simulink model "IEEE_9bus_v2_"  (Simulink 8.4)
settings: Solver=ode4  StartTime=0.0  StopTime=inf  FixedStep=Ts  RelTol=1e-3
PostLoadFcn:
  | Ts=25e-6;Rs=5*1.867;cs=1.4080e-004;
InitFcn:
  | Ts=25e-6;Rs=5*1.867;cs=1.4080e-004;
undefined symbols (not defined in the file): another_event_name, DiscIntNeverNeededParam, gcbh, my_event_name, sps_rtmsupport
libraries: powerlib x36, spsVIMeasurementModel x27, library x9, rtlab x4, artemis x3, sps_avr x3
(part 2 of 2)

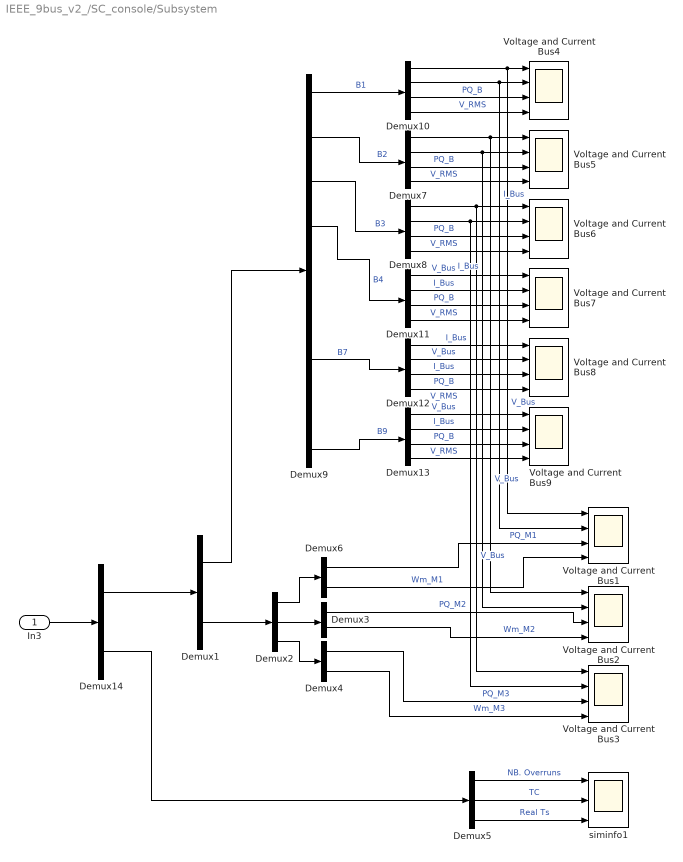
== system IEEE_9bus_v2_/SC_console/Subsystem ==
  In3 : Inport
  Demux1 : Demux  Outputs=[99 9]
  Demux{7..8,10..13} (6 alike) : Demux  Outputs=[3 3 2 3]
  Demux14 : Demux  Outputs=[108 3]
  Demux2 : Demux  Outputs=3
  Demux3 : Demux  Outputs=[2 1]
  Demux4 : Demux  Outputs=[2 1]
  Demux5 : Demux  Outputs=3
  Demux6 : Demux  Outputs=[2 1]
  Demux9 : Demux  Outputs=[11 11 11 11 11 11 11 11 11]
  Voltage and Current Bus{1..9} (9 alike) : Scope  NumInputPorts=4
      Voltage and Current Bus1 settings: TimeRange=0.1  MaxDataPoints=15000  SaveToWorkspace=off  SaveName=mach10  YMin=-1.25~-0.75~-0.5~1  YMax=1.25~0.75~0.3~1.00001  SampleTime=-1
      Voltage and Current Bus2 settings: TimeRange=0.1  MaxDataPoints=15000  SaveToWorkspace=off  SaveName=mach11  YMin=-1.25~-0.75~-0.5~1  YMax=1.25~0.75~0.3~1.00001  SampleTime=-1
      Voltage and Current Bus3 settings: TimeRange=0.1  MaxDataPoints=15000  SaveToWorkspace=off  SaveName=mach12  YMin=-1.25~-0.75~-0.5~1  YMax=1.25~0.75~0.3~1.00001  SampleTime=-1
      Voltage and Current Bus4 settings: TimeRange=0.1  LimitDataPoints=on  MaxDataPoints=15000  SaveToWorkspace=off  SaveName=mach13  YMin=-1~-0.9~-0.8~-5  YMax=1~0.9~0.5~5  SampleTime=-1
      Voltage and Current Bus5 settings: TimeRange=0.1  LimitDataPoints=on  MaxDataPoints=15000  SaveToWorkspace=off  SaveName=mach  YMin=-1~-0.9~-0.8~-5  YMax=1~0.9~0.5~5  SampleTime=-1
      Voltage and Current Bus6 settings: TimeRange=0.1  LimitDataPoints=on  MaxDataPoints=15000  SaveToWorkspace=off  SaveName=mach1  YMin=-1~-0.9~-0.8~-5  YMax=1~0.9~0.5~5  SampleTime=-1
      Voltage and Current Bus7 settings: TimeRange=0.1  LimitDataPoints=on  MaxDataPoints=15000  SaveToWorkspace=off  SaveName=mach3  YMin=-1~-0.9~-0.8~-5  YMax=1~0.9~0.5~5  SampleTime=-1
      Voltage and Current Bus8 settings: TimeRange=0.1  LimitDataPoints=on  MaxDataPoints=15000  SaveToWorkspace=off  SaveName=mach4  YMin=-1~-0.9~-0.8~-5  YMax=1~0.9~0.5~5  SampleTime=-1
      Voltage and Current Bus9 settings: TimeRange=0.1  LimitDataPoints=on  MaxDataPoints=15000  SaveToWorkspace=off  SaveName=mach5  YMin=-1~-0.9~-0.8~-5  YMax=1~0.9~0.5~5  SampleTime=-1
  siminfo1 : Scope  NumInputPorts=3
      settings: TimeRange=0.8  LimitDataPoints=on  MaxDataPoints=15000  SaveToWorkspace=off  SaveName=mach2  YMin=-1~-1~-1  YMax=1~1~1  SampleTime=-1
  wires:
  Demux5/3 -> siminfo1/3  "Real Ts"
  Demux5/1 -> siminfo1/1  "NB. Overruns"
  Demux5/2 -> siminfo1/2  "TC"
  Demux3/2 -> Voltage and Current Bus2/4  "Wm_M2"
  Demux2/1 -> Demux6/1
  Demux6/1 -> Voltage and Current Bus1/3  "PQ_M1"
  Demux1/2 -> Demux2/1
  Demux4/2 -> Voltage and Current Bus3/4  "Wm_M3"
  Demux4/1 -> Voltage and Current Bus3/3  "PQ_M3"
  Demux3/1 -> Voltage and Current Bus2/3  "PQ_M2"
  Demux2/2 -> Demux3/1
  Demux2/3 -> Demux4/1
  Demux6/2 -> Voltage and Current Bus1/4  "Wm_M1"
  Demux1/1 -> Demux9/1
  Demux9/1 -> Demux10/1  "B1"
  Demux10/1 -> Voltage and Current Bus1/1, Voltage and Current Bus4/1  "V_Bus"
  Demux10/2 -> Voltage and Current Bus1/2, Voltage and Current Bus4/2  "I_Bus"
  Demux10/3 -> Voltage and Current Bus4/3  "PQ_B"
  In3/1 -> Demux14/1
  Demux14/2 -> Demux5/1
  Demux14/1 -> Demux1/1
  Demux10/4 -> Voltage and Current Bus4/4  "V_RMS"
  Demux7/1 -> Voltage and Current Bus2/1, Voltage and Current Bus5/1  "V_Bus"
  Demux7/2 -> Voltage and Current Bus2/2, Voltage and Current Bus5/2  "I_Bus"
  Demux7/3 -> Voltage and Current Bus5/3  "PQ_B"
  Demux7/4 -> Voltage and Current Bus5/4  "V_RMS"
  Demux8/1 -> Voltage and Current Bus3/1, Voltage and Current Bus6/1  "V_Bus"
  Demux8/2 -> Voltage and Current Bus3/2, Voltage and Current Bus6/2  "I_Bus"
  Demux8/3 -> Voltage and Current Bus6/3  "PQ_B"
  Demux8/4 -> Voltage and Current Bus6/4  "V_RMS"
  Demux11/1 -> Voltage and Current Bus7/1  "V_Bus"
  Demux11/2 -> Voltage and Current Bus7/2  "I_Bus"
  Demux11/3 -> Voltage and Current Bus7/3  "PQ_B"
  Demux11/4 -> Voltage and Current Bus7/4  "V_RMS"
  Demux12/1 -> Voltage and Current Bus8/1  "V_Bus"
  Demux12/2 -> Voltage and Current Bus8/2  "I_Bus"
  Demux12/3 -> Voltage and Current Bus8/3  "PQ_B"
  Demux12/4 -> Voltage and Current Bus8/4  "V_RMS"
  Demux13/1 -> Voltage and Current Bus9/1  "V_Bus"
  Demux13/2 -> Voltage and Current Bus9/2  "I_Bus"
  Demux13/3 -> Voltage and Current Bus9/3  "PQ_B"
  Demux13/4 -> Voltage and Current Bus9/4  "V_RMS"
  Demux9/2 -> Demux7/1  "B2"
  Demux9/3 -> Demux8/1  "B3"
  Demux9/4 -> Demux11/1  "B4"
  Demux9/7 -> Demux12/1  "B7"
  Demux9/9 -> Demux13/1  "B9"

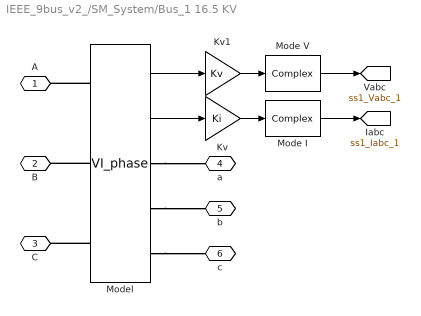
== system IEEE_9bus_v2_/SM_System/Bus_1 16.5 KV ==
  Kv : Gain  Gain=Ki  SaturateOnIntegerOverflow=on  OutDataTypeStr=Inherit: Same as input  ParamDataTypeStr=Inherit: Same as input
  Kv1 : Gain  Gain=Kv  SaturateOnIntegerOverflow=on  OutDataTypeStr=Inherit: Same as input  ParamDataTypeStr=Inherit: Same as input
  Mode I : spsVIMeasurementModel/Complex
  Mode V : spsVIMeasurementModel/Complex
  Model : spsVIMeasurementModel/VI_phase  SystemSampleTime=-1
  A : PMIOPort  Port=1  Side=Left
  B : PMIOPort  Port=2  Side=Left
  C : PMIOPort  Port=3  Side=Left
  a : PMIOPort  Port=4  Side=Right
  b : PMIOPort  Port=5  Side=Right
  c : PMIOPort  Port=6  Side=Right
  tag scope: ss1_Iabc_1=global, ss1_Vabc_1=global
  wires:
  Model/2 -> Kv/1
  Model/1 -> Kv1/1
  Kv/1 -> Mode I/1
  Kv1/1 -> Mode V/1
  Mode I/1 -> [ss1_Iabc_1]
  Mode V/1 -> [ss1_Vabc_1]
  connections:
  Model/RConn3 -- c/RConn1
  Model/RConn1 -- a/RConn1
  Model/RConn2 -- b/RConn1
  Model/LConn3 -- C/RConn1
  Model/LConn1 -- A/RConn1
  Model/LConn2 -- B/RConn1

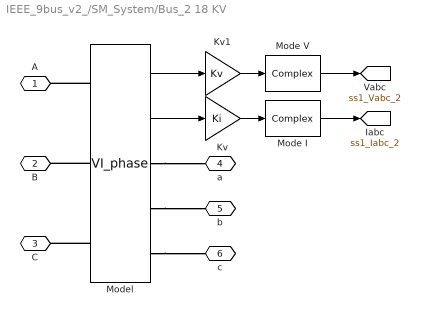
== system IEEE_9bus_v2_/SM_System/Bus_2 18 KV ==
  Kv : Gain  Gain=Ki  SaturateOnIntegerOverflow=on  OutDataTypeStr=Inherit: Same as input  ParamDataTypeStr=Inherit: Same as input
  Kv1 : Gain  Gain=Kv  SaturateOnIntegerOverflow=on  OutDataTypeStr=Inherit: Same as input  ParamDataTypeStr=Inherit: Same as input
  Mode I : spsVIMeasurementModel/Complex
  Mode V : spsVIMeasurementModel/Complex
  Model : spsVIMeasurementModel/VI_phase  SystemSampleTime=-1
  A : PMIOPort  Port=1  Side=Left
  B : PMIOPort  Port=2  Side=Left
  C : PMIOPort  Port=3  Side=Left
  a : PMIOPort  Port=4  Side=Right
  b : PMIOPort  Port=5  Side=Right
  c : PMIOPort  Port=6  Side=Right
  tag scope: ss1_Iabc_2=global, ss1_Vabc_2=global
  wires:
  Model/2 -> Kv/1
  Model/1 -> Kv1/1
  Kv/1 -> Mode I/1
  Kv1/1 -> Mode V/1
  Mode I/1 -> [ss1_Iabc_2]
  Mode V/1 -> [ss1_Vabc_2]
  connections:
  Model/RConn3 -- c/RConn1
  Model/RConn1 -- a/RConn1
  Model/RConn2 -- b/RConn1
  Model/LConn3 -- C/RConn1
  Model/LConn1 -- A/RConn1
  Model/LConn2 -- B/RConn1

== system IEEE_9bus_v2_/SM_System/Bus_3 13.8 KV ==
  Kv : Gain  Gain=Ki  SaturateOnIntegerOverflow=on  OutDataTypeStr=Inherit: Same as input  ParamDataTypeStr=Inherit: Same as input
  Kv1 : Gain  Gain=Kv  SaturateOnIntegerOverflow=on  OutDataTypeStr=Inherit: Same as input  ParamDataTypeStr=Inherit: Same as input
  Mode I : spsVIMeasurementModel/Complex
  Mode V : spsVIMeasurementModel/Complex
  Model : spsVIMeasurementModel/VI_phase  SystemSampleTime=-1
  A : PMIOPort  Port=1  Side=Left
  B : PMIOPort  Port=2  Side=Left
  C : PMIOPort  Port=3  Side=Left
  a : PMIOPort  Port=4  Side=Right
  b : PMIOPort  Port=5  Side=Right
  c : PMIOPort  Port=6  Side=Right
  tag scope: ss1_Iabc_3=global, ss1_Vabc_3=global
  wires:
  Model/2 -> Kv/1
  Model/1 -> Kv1/1
  Kv/1 -> Mode I/1
  Kv1/1 -> Mode V/1
  Mode I/1 -> [ss1_Iabc_3]
  Mode V/1 -> [ss1_Vabc_3]
  connections:
  Model/RConn3 -- c/RConn1
  Model/RConn1 -- a/RConn1
  Model/RConn2 -- b/RConn1
  Model/LConn3 -- C/RConn1
  Model/LConn1 -- A/RConn1
  Model/LConn2 -- B/RConn1

== system IEEE_9bus_v2_/SM_System/Bus_4 230 KV ==
  Kv : Gain  Gain=Ki  SaturateOnIntegerOverflow=on  OutDataTypeStr=Inherit: Same as input  ParamDataTypeStr=Inherit: Same as input
  Kv1 : Gain  Gain=Kv  SaturateOnIntegerOverflow=on  OutDataTypeStr=Inherit: Same as input  ParamDataTypeStr=Inherit: Same as input
  Mode I : spsVIMeasurementModel/Complex
  Mode V : spsVIMeasurementModel/Complex
  Model : spsVIMeasurementModel/VI_phase  SystemSampleTime=-1
  A : PMIOPort  Port=1  Side=Left
  B : PMIOPort  Port=2  Side=Left
  C : PMIOPort  Port=3  Side=Left
  a : PMIOPort  Port=4  Side=Right
  b : PMIOPort  Port=5  Side=Right
  c : PMIOPort  Port=6  Side=Right
  tag scope: ss1_Iabc_4=global, ss1_Vabc_4=global
  wires:
  Model/2 -> Kv/1
  Model/1 -> Kv1/1
  Kv/1 -> Mode I/1
  Kv1/1 -> Mode V/1
  Mode I/1 -> [ss1_Iabc_4]
  Mode V/1 -> [ss1_Vabc_4]
  connections:
  Model/RConn3 -- c/RConn1
  Model/RConn1 -- a/RConn1
  Model/RConn2 -- b/RConn1
  Model/LConn3 -- C/RConn1
  Model/LConn1 -- A/RConn1
  Model/LConn2 -- B/RConn1

== system IEEE_9bus_v2_/SM_System/Bus_5 230 KV ==
  Kv : Gain  Gain=Ki  SaturateOnIntegerOverflow=on  OutDataTypeStr=Inherit: Same as input  ParamDataTypeStr=Inherit: Same as input
  Kv1 : Gain  Gain=Kv  SaturateOnIntegerOverflow=on  OutDataTypeStr=Inherit: Same as input  ParamDataTypeStr=Inherit: Same as input
  Mode I : spsVIMeasurementModel/Complex
  Mode V : spsVIMeasurementModel/Complex
  Model : spsVIMeasurementModel/VI_phase  SystemSampleTime=-1
  A : PMIOPort  Port=1  Side=Left
  B : PMIOPort  Port=2  Side=Left
  C : PMIOPort  Port=3  Side=Left
  a : PMIOPort  Port=4  Side=Right
  b : PMIOPort  Port=5  Side=Right
  c : PMIOPort  Port=6  Side=Right
  tag scope: ss1_Iabc_5=global, ss1_Vabc_5=global
  wires:
  Model/2 -> Kv/1
  Model/1 -> Kv1/1
  Kv/1 -> Mode I/1
  Kv1/1 -> Mode V/1
  Mode I/1 -> [ss1_Iabc_5]
  Mode V/1 -> [ss1_Vabc_5]
  connections:
  Model/RConn3 -- c/RConn1
  Model/RConn1 -- a/RConn1
  Model/RConn2 -- b/RConn1
  Model/LConn3 -- C/RConn1
  Model/LConn1 -- A/RConn1
  Model/LConn2 -- B/RConn1

== system IEEE_9bus_v2_/SM_System/Bus_6 230 KV ==
  Kv : Gain  Gain=Ki  SaturateOnIntegerOverflow=on  OutDataTypeStr=Inherit: Same as input  ParamDataTypeStr=Inherit: Same as input
  Kv1 : Gain  Gain=Kv  SaturateOnIntegerOverflow=on  OutDataTypeStr=Inherit: Same as input  ParamDataTypeStr=Inherit: Same as input
  Mode I : spsVIMeasurementModel/Complex
  Mode V : spsVIMeasurementModel/Complex
  Model : spsVIMeasurementModel/VI_phase  SystemSampleTime=-1
  A : PMIOPort  Port=1  Side=Left
  B : PMIOPort  Port=2  Side=Left
  C : PMIOPort  Port=3  Side=Left
  a : PMIOPort  Port=4  Side=Right
  b : PMIOPort  Port=5  Side=Right
  c : PMIOPort  Port=6  Side=Right
  tag scope: ss1_Iabc_6=global, ss1_Vabc_6=global
  wires:
  Model/2 -> Kv/1
  Model/1 -> Kv1/1
  Kv/1 -> Mode I/1
  Kv1/1 -> Mode V/1
  Mode I/1 -> [ss1_Iabc_6]
  Mode V/1 -> [ss1_Vabc_6]
  connections:
  Model/RConn3 -- c/RConn1
  Model/RConn1 -- a/RConn1
  Model/RConn2 -- b/RConn1
  Model/LConn3 -- C/RConn1
  Model/LConn1 -- A/RConn1
  Model/LConn2 -- B/RConn1

== system IEEE_9bus_v2_/SM_System/Bus_7 230 KV  ==
  Kv : Gain  Gain=Ki  SaturateOnIntegerOverflow=on  OutDataTypeStr=Inherit: Same as input  ParamDataTypeStr=Inherit: Same as input
  Kv1 : Gain  Gain=Kv  SaturateOnIntegerOverflow=on  OutDataTypeStr=Inherit: Same as input  ParamDataTypeStr=Inherit: Same as input
  Mode I : spsVIMeasurementModel/Complex
  Mode V : spsVIMeasurementModel/Complex
  Model : spsVIMeasurementModel/VI_phase  SystemSampleTime=-1
  A : PMIOPort  Port=1  Side=Left
  B : PMIOPort  Port=2  Side=Left
  C : PMIOPort  Port=3  Side=Left
  a : PMIOPort  Port=4  Side=Right
  b : PMIOPort  Port=5  Side=Right
  c : PMIOPort  Port=6  Side=Right
  tag scope: ss1_Iabc_7=global, ss1_Vabc_7=global
  wires:
  Model/2 -> Kv/1
  Model/1 -> Kv1/1
  Kv/1 -> Mode I/1
  Kv1/1 -> Mode V/1
  Mode I/1 -> [ss1_Iabc_7]
  Mode V/1 -> [ss1_Vabc_7]
  connections:
  Model/RConn3 -- c/RConn1
  Model/RConn1 -- a/RConn1
  Model/RConn2 -- b/RConn1
  Model/LConn3 -- C/RConn1
  Model/LConn1 -- A/RConn1
  Model/LConn2 -- B/RConn1

== system IEEE_9bus_v2_/SM_System/Bus_8 230 KV ==
  Kv : Gain  Gain=Ki  SaturateOnIntegerOverflow=on  OutDataTypeStr=Inherit: Same as input  ParamDataTypeStr=Inherit: Same as input
  Kv1 : Gain  Gain=Kv  SaturateOnIntegerOverflow=on  OutDataTypeStr=Inherit: Same as input  ParamDataTypeStr=Inherit: Same as input
  Mode I : spsVIMeasurementModel/Complex
  Mode V : spsVIMeasurementModel/Complex
  Model : spsVIMeasurementModel/VI_phase  SystemSampleTime=-1
  A : PMIOPort  Port=1  Side=Left
  B : PMIOPort  Port=2  Side=Left
  C : PMIOPort  Port=3  Side=Left
  a : PMIOPort  Port=4  Side=Right
  b : PMIOPort  Port=5  Side=Right
  c : PMIOPort  Port=6  Side=Right
  tag scope: ss1_Iabc_8=global, ss1_Vabc_8=global
  wires:
  Model/2 -> Kv/1
  Model/1 -> Kv1/1
  Kv/1 -> Mode I/1
  Kv1/1 -> Mode V/1
  Mode I/1 -> [ss1_Iabc_8]
  Mode V/1 -> [ss1_Vabc_8]
  connections:
  Model/RConn3 -- c/RConn1
  Model/RConn1 -- a/RConn1
  Model/RConn2 -- b/RConn1
  Model/LConn3 -- C/RConn1
  Model/LConn1 -- A/RConn1
  Model/LConn2 -- B/RConn1

== system IEEE_9bus_v2_/SM_System/Bus_9 230 KV ==
  Kv : Gain  Gain=Ki  SaturateOnIntegerOverflow=on  OutDataTypeStr=Inherit: Same as input  ParamDataTypeStr=Inherit: Same as input
  Kv1 : Gain  Gain=Kv  SaturateOnIntegerOverflow=on  OutDataTypeStr=Inherit: Same as input  ParamDataTypeStr=Inherit: Same as input
  Mode I : spsVIMeasurementModel/Complex
  Mode V : spsVIMeasurementModel/Complex
  Model : spsVIMeasurementModel/VI_phase  SystemSampleTime=-1
  A : PMIOPort  Port=1  Side=Left
  B : PMIOPort  Port=2  Side=Left
  C : PMIOPort  Port=3  Side=Left
  a : PMIOPort  Port=4  Side=Right
  b : PMIOPort  Port=5  Side=Right
  c : PMIOPort  Port=6  Side=Right
  tag scope: ss1_Iabc_9=global, ss1_Vabc_9=global
  wires:
  Model/2 -> Kv/1
  Model/1 -> Kv1/1
  Kv/1 -> Mode I/1
  Kv1/1 -> Mode V/1
  Mode I/1 -> [ss1_Iabc_9]
  Mode V/1 -> [ss1_Vabc_9]
  connections:
  Model/RConn3 -- c/RConn1
  Model/RConn1 -- a/RConn1
  Model/RConn2 -- b/RConn1
  Model/LConn3 -- C/RConn1
  Model/LConn1 -- A/RConn1
  Model/LConn2 -- B/RConn1

== system IEEE_9bus_v2_/SM_System/Fault_Gen ==
  In1 : Inport
  Constant1 : Constant  Value=[0 0]  SampleTime=-1
  Demux4 : Demux  Outputs=[1 3 3 1 1 1 1]
  Sine Wave : Sin  Frequency=2*pi*60  SampleTime=Ts
  faultgen : Subsystem
  Fault : Outport
  Pert : Outport  Port=2
  TTigger : Outport  Port=3
  tag scope: L1=global, L2=global, L3=global, fault_type=global
  wires:
  Sine Wave/1 -> faultgen/6(pulse)
  Constant1/1 -> faultgen/5(pert_set)
  Demux4/1 -> faultgen/1(Tacq)
  Demux4/2 -> faultgen/2(Tst_set)
  Demux4/3 -> faultgen/3(Tdr_set)
  Demux4/4 -> faultgen/4(faultype), [fault_type]
  Demux4/5 -> [L1]
  faultgen/1(fault) -> Fault/1
  In1/1 -> Demux4/1
  faultgen/2(pertb) -> Pert/1
  faultgen/3(trig) -> TTigger/1
  Demux4/6 -> [L2]
  Demux4/7 -> [L3]

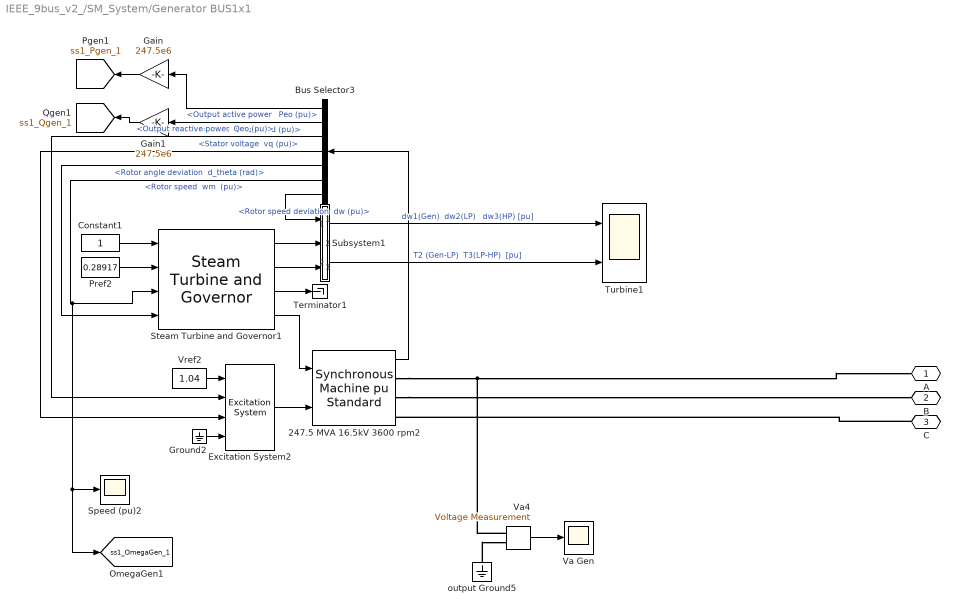
== system IEEE_9bus_v2_/SM_System/Generator BUS1x1 ==
  " Speed (pu)2" : Scope
      settings: TimeRange=100  TickLabels=on  MaxDataPoints=5000  SaveName=ss1_Gen1Freq  YMin=0.995  YMax=1  SampleTime=-1
  247.5 MVA 16.5kV 3600 rpm2 : powerlib/Machines/Synchronous Machine pu Standard  PresetModel=No  MechanicalLoad=Mechanical power Pm  ShowDetailedParameters=on  RotorType=Round  Units=per unit standard parameters  MeasurementBus=off  NominalParameters="[ 247.5e6  16.5e3   60 ]"  Reactances1=[ 0.36135, 0.15048, 0.12375, 0.2475, 0.2398275, 0.12375, 0.08316 ]  Reactances2="[ 1.305, 0.296, 0.252, 0.474,  0.243,  0.18 ]"  dAxisTimeConstants=Open-circuit  qAxisTimeConstants=Open-circuit  TimeConstants1="[ 4.4849  0.0681  0.1  ]"  TimeConstants2="[ 8.96, 0.05,  0.31, 0.05 ]"  TimeConstants3="[  4.49  0.0681  0.0513  ]"  TimeConstants4=[ 8.0, 0.03, 0.3371, 0.0295 ]  TimeConstants5=[ 1.01, 0.053, 0.1 ]  TimeConstants6=[ 1.3201, 0.023, 1.0, 0.07 ]  TimeConstants7="[  1.01  0.053  0.051266  ]"  TimeConstants8=[ 1.3201, 0.0231, 0.3371, 0.0295 ]  StatorResistance=0.000125  Mechanical="[ 23.64  0 1 ]"  PolePairs=1  InitialConditions=[0 -86.3058 0.296671 0.296671 0.296671 -20.4087 -140.409 99.5913 1.08165]  SetSaturation=off  Saturation=[0.6404,0.7127,0.8441,0.9214,0.9956,1.082,1.19,1.316,1.457;0.7,0.7698,0.8872,0.9466,0.9969,1.046,1.1,1.151,1.201]  LoadFlowParameters=[2 71600000 0 0 0]  TsPowergui=0  TsBlock=-1  IterativeModel=Trapezoidal non iterative  IterativeDiscreteModel=Trapezoidal non iterative  BusType=swing  Pref=0  Qref=0  Qmin=-Inf  Qmax=Inf  PLF=0  QLF=0
  Bus Selector3 : BusSelector  OutputSignals="Output active power   Peo (pu),Output reactive power  Qeo (pu),dq0 components.Stator voltage  vd (pu),dq0 components.Stator voltage  vq (pu),Mechanical.Rotor angle deviation  d_theta (rad),Mechanical.Rotor speed  wm  (pu),Mechanical.Rotor speed deviation  dw (pu)"
  Constant1 : Constant
  Excitation System2 : sps_avr/Excitation System  tr=20e-3  reg=[ 200, 0.02 ]  exc=[ 1, 0 ]  tgr=[ 12.0, 1.0 ]  damp=[ 0.03, 1.0 ]  sat=[ 0, 0 ]  lim=[ -10.0, 10.0, 0 ]  v0=[1.04 1.0817]
  Gain : Gain  Gain=247.5e6
  Gain1 : Gain  Gain=247.5e6
  Ground2 : Ground
  Pref2 : Constant  Value=0.28917
  Steam Turbine and Governor1 : powerlib/Machines/Steam Turbine and Governor  gentype=Tandem-compound (single mass)  reg1="[ 1  0.05    0 ]"  reg2="[ 0.001  0.1 ]"  reg3="[ -10.0 0.1   0.1 1.0 ]"  N=3600  turb1="[ 0.12  0.13  10.0   0.32   ]"  turb2="[ 0.48   0.25   0  0.27 ]"  HA="[  1.5498   0.24894  0  0 ]"  KA="[  83.47  42.702  0  0 ]"  DA="[  0.3104  0.05  0  0 ]*8"  ini1=0.28918  ini2=[1.88924e-008,-120.067]
  Subsystem1 : Subsystem
  Terminator1 : Terminator
  Turbine1 : Scope  NumInputPorts=2
      settings: TimeRange=0.5  MaxDataPoints=5000  SaveToWorkspace=off  SaveName=ss1_ScopeData2  YMin=0~-1  YMax=3e+09~1  SampleTime=-1
  Va Gen : Scope
      settings: TimeRange=2  TickLabels=on  MaxDataPoints=5000  SaveToWorkspace=off  SaveName=ss1_vf4  YMin=-15000  YMax=15000  SampleTime=-1  DataFormat=Array
  Va4 : powerlib/Measurements/Voltage Measurement  Tag=PoWeRsYsTeMmEaSuReMeNt  PhasorSimulation=off  OutputType=Magnitude  PSBequivalent=0
  Vref2 : Constant  Value=1.04
  output Ground5 : powerlib/Elements/Ground  LConnTagsString=a
  A : PMIOPort  Port=1  Side=Right
  B : PMIOPort  Port=2  Side=Right
  C : PMIOPort  Port=3  Side=Right
  tag scope: ss1_OmegaGen_1=global, ss1_Pgen_1=global, ss1_Qgen_1=global
  wires:
  Constant1/1 -> Steam Turbine and Governor1/1
  Bus Selector3/5 -> Steam Turbine and Governor1/4  "<Rotor angle deviation  d_theta (rad)>"
  Subsystem1/2(T_23) -> Turbine1/2  "T2 (Gen-LP)  T3(LP-HP)  [pu]"
  Steam Turbine and Governor1/3 -> Terminator1/1
  Bus Selector3/7 -> Subsystem1/1(In1)  "<Rotor speed deviation  dw (pu)>"
  Vref2/1 -> Excitation System2/1
  Pref2/1 -> Steam Turbine and Governor1/2
  Steam Turbine and Governor1/1 -> Subsystem1/2(In2)
  Subsystem1/1(dw_123) -> Turbine1/1  "dw1(Gen)  dw2(LP)   dw3(HP) [pu]"
  Steam Turbine and Governor1/4 -> 247.5 MVA 16.5kV 3600 rpm2/1
  Steam Turbine and Governor1/2 -> Subsystem1/3(In3)
  Bus Selector3/6 -> [ss1_OmegaGen_1], " Speed (pu)2"/1, Steam Turbine and Governor1/3  "<Rotor speed  wm  (pu)>"
  247.5 MVA 16.5kV 3600 rpm2/1 -> Bus Selector3/1
  Ground2/1 -> Excitation System2/4
  Bus Selector3/4 -> Excitation System2/3  "<Stator voltage  vq (pu)>"
  Bus Selector3/3 -> Excitation System2/2  "<Stator voltage  vd (pu)>"
  Excitation System2/1 -> 247.5 MVA 16.5kV 3600 rpm2/2
  Va4/1 -> Va Gen/1
  Bus Selector3/1 -> Gain/1  "<Output active power   Peo (pu)>"
  Bus Selector3/2 -> Gain1/1  "<Output reactive power  Qeo (pu)>"
  Gain/1 -> [ss1_Pgen_1]
  Gain1/1 -> [ss1_Qgen_1]
  connections:
  output Ground5/LConn1 -- Va4/LConn2
  C/RConn1 -- 247.5 MVA 16.5kV 3600 rpm2/RConn3
  247.5 MVA 16.5kV 3600 rpm2/RConn2 -- B/RConn1
  Va4/LConn1 -- 247.5 MVA 16.5kV 3600 rpm2/RConn1 -- A/RConn1

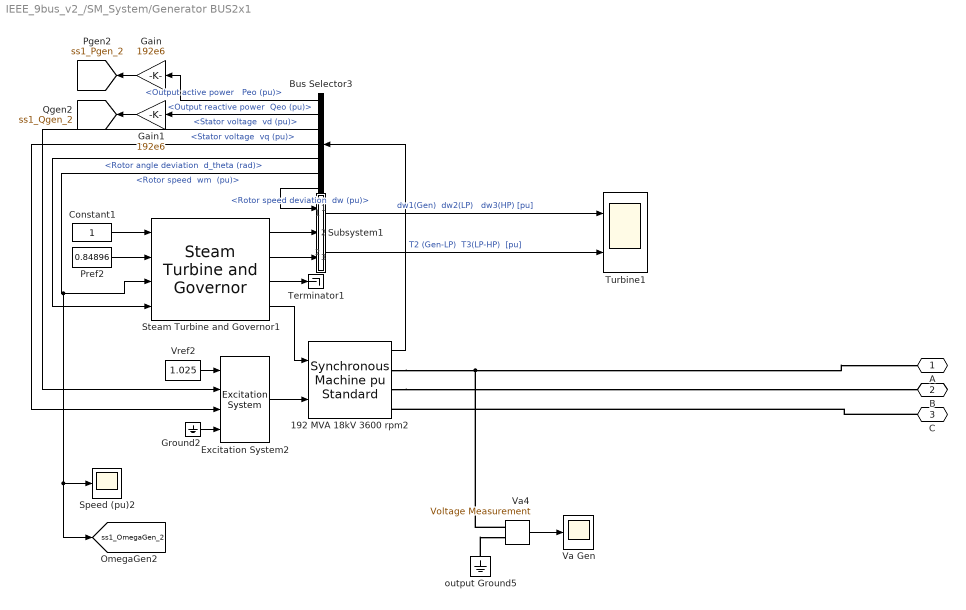
== system IEEE_9bus_v2_/SM_System/Generator BUS2x1 ==
  " Speed (pu)2" : Scope
      settings: TimeRange=150  TickLabels=on  MaxDataPoints=5000  SaveToWorkspace=off  SaveName=ss1_Pm2  YMin=0.995  YMax=1  SampleTime=-1  DataFormat=Array
  192 MVA 18kV 3600 rpm2 : powerlib/Machines/Synchronous Machine pu Standard  PresetModel=No  MechanicalLoad=Mechanical power Pm  ShowDetailedParameters=on  RotorType=Round  Units=per unit standard parameters  MeasurementBus=off  NominalParameters="[ 192e6  18e3   60 ]"  Reactances1=[ 1.719936, 0.230016, 0.1632, 1.65984, 0.378048, 0.2304, 0.10002 ]  Reactances2="[ 1.305, 0.296, 0.252, 0.474,  0.243,  0.18 ]"  dAxisTimeConstants=Open-circuit  qAxisTimeConstants=Open-circuit  TimeConstants1="[ 4.4849  0.0681  0.1  ]"  TimeConstants2="[ 6.0, 0.05,  0.535, 0.05 ]"  TimeConstants3="[  4.49  0.0681  0.0513  ]"  TimeConstants4=[ 8.0, 0.03, 0.3371, 0.0295 ]  TimeConstants5=[ 1.01, 0.053, 0.1 ]  TimeConstants6=[ 1.3201, 0.023, 1.0, 0.07 ]  TimeConstants7="[  1.01  0.053  0.051266  ]"  TimeConstants8=[ 1.3201, 0.0231, 0.3371, 0.0295 ]  StatorResistance=0.000125  Mechanical="[ 6.4  0 1 ]"  PolePairs=1  InitialConditions=[0 -28.9349 0.828916 0.828916 0.828916 6.92884 -113.071 126.929 1.78871]  SetSaturation=off  Saturation=[0.6404,0.7127,0.8441,0.9214,0.9956,1.082,1.19,1.316,1.457;0.7,0.7698,0.8872,0.9466,0.9969,1.046,1.1,1.151,1.201]  LoadFlowParameters=[1 163000000 0 0 0]  TsPowergui=0  TsBlock=-1  IterativeModel=Trapezoidal non iterative  IterativeDiscreteModel=Trapezoidal non iterative  BusType=PV  Pref=163e6  Qref=0  Qmin=-Inf  Qmax=Inf  PLF=0  QLF=0
  Bus Selector3 : BusSelector  OutputSignals="Output active power   Peo (pu),Output reactive power  Qeo (pu),dq0 components.Stator voltage  vd (pu),dq0 components.Stator voltage  vq (pu),Mechanical.Rotor angle deviation  d_theta (rad),Mechanical.Rotor speed  wm  (pu),Mechanical.Rotor speed deviation  dw (pu)"
  Constant1 : Constant
  Excitation System2 : sps_avr/Excitation System  tr=20e-3  reg=[ 200, 0.02 ]  exc=[ 1, 0 ]  tgr=[ 12.0, 1.0 ]  damp=[ 0.03, 1.0 ]  sat=[ 0, 0 ]  lim=[ -10.0, 10.0, 0 ]  v0=[1.025 1.7887]
  Gain : Gain  Gain=192e6
  Gain1 : Gain  Gain=192e6
  Ground2 : Ground
  Pref2 : Constant  Value=0.84896
  Steam Turbine and Governor1 : powerlib/Machines/Steam Turbine and Governor  gentype=Tandem-compound (single mass)  reg1="[ 1  0.05    0 ]"  reg2="[ 0.001  0.1 ]"  reg3="[ -10.0 0.1   0.1 1.0 ]"  N=3600  turb1="[ 0.12  0.13  10.0   0.32   ]"  turb2="[ 0.48   0.25   0  0.27 ]"  HA="[  1.5498   0.24894  0  0 ]"  KA="[  83.47  42.702  0  0 ]"  DA="[  0.3104  0.05  0  0 ]*8"  ini1=0.84904  ini2=[1.88924e-008,-120.067]
  Subsystem1 : Subsystem
  Terminator1 : Terminator
  Turbine1 : Scope  NumInputPorts=2
      settings: TimeRange=0.5  MaxDataPoints=5000  SaveToWorkspace=off  SaveName=ss1_ScopeData2  YMin=-0.03~-5  YMax=0.03~5  SampleTime=-1
  Va Gen : Scope
      settings: TimeRange=150  TickLabels=on  MaxDataPoints=5000  SaveToWorkspace=off  SaveName=ss1_vf4  YMin=-20000  YMax=20000  SampleTime=-1  DataFormat=Array
  Va4 : powerlib/Measurements/Voltage Measurement  Tag=PoWeRsYsTeMmEaSuReMeNt  PhasorSimulation=off  OutputType=Magnitude  PSBequivalent=0
  Vref2 : Constant  Value=1.025
  output Ground5 : powerlib/Elements/Ground  LConnTagsString=a
  A : PMIOPort  Port=1  Side=Right
  B : PMIOPort  Port=2  Side=Right
  C : PMIOPort  Port=3  Side=Right
  tag scope: ss1_OmegaGen_2=global, ss1_Pgen_2=global, ss1_Qgen_2=global
  wires:
  Constant1/1 -> Steam Turbine and Governor1/1
  Bus Selector3/5 -> Steam Turbine and Governor1/4  "<Rotor angle deviation  d_theta (rad)>"
  Subsystem1/2(T_23) -> Turbine1/2  "T2 (Gen-LP)  T3(LP-HP)  [pu]"
  Steam Turbine and Governor1/3 -> Terminator1/1
  Bus Selector3/7 -> Subsystem1/1(In1)  "<Rotor speed deviation  dw (pu)>"
  Vref2/1 -> Excitation System2/1
  Pref2/1 -> Steam Turbine and Governor1/2
  Steam Turbine and Governor1/1 -> Subsystem1/2(In2)
  Subsystem1/1(dw_123) -> Turbine1/1  "dw1(Gen)  dw2(LP)   dw3(HP) [pu]"
  Steam Turbine and Governor1/4 -> 192 MVA 18kV 3600 rpm2/1
  Steam Turbine and Governor1/2 -> Subsystem1/3(In3)
  Bus Selector3/6 -> [ss1_OmegaGen_2], " Speed (pu)2"/1, Steam Turbine and Governor1/3  "<Rotor speed  wm  (pu)>"
  192 MVA 18kV 3600 rpm2/1 -> Bus Selector3/1
  Ground2/1 -> Excitation System2/4
  Bus Selector3/4 -> Excitation System2/3  "<Stator voltage  vq (pu)>"
  Bus Selector3/3 -> Excitation System2/2  "<Stator voltage  vd (pu)>"
  Excitation System2/1 -> 192 MVA 18kV 3600 rpm2/2
  Va4/1 -> Va Gen/1
  Bus Selector3/2 -> Gain1/1  "<Output reactive power  Qeo (pu)>"
  Bus Selector3/1 -> Gain/1  "<Output active power   Peo (pu)>"
  Gain/1 -> [ss1_Pgen_2]
  Gain1/1 -> [ss1_Qgen_2]
  connections:
  output Ground5/LConn1 -- Va4/LConn2
  C/RConn1 -- 192 MVA 18kV 3600 rpm2/RConn3
  192 MVA 18kV 3600 rpm2/RConn2 -- B/RConn1
  Va4/LConn1 -- 192 MVA 18kV 3600 rpm2/RConn1 -- A/RConn1

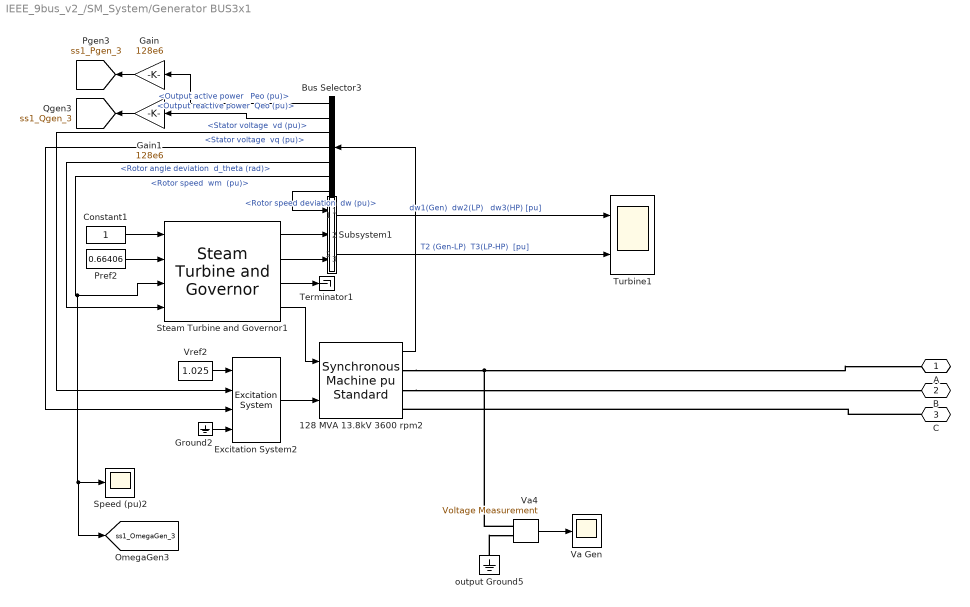
== system IEEE_9bus_v2_/SM_System/Generator BUS3x1 ==
  " Speed (pu)2" : Scope
      settings: TimeRange=150  TickLabels=on  MaxDataPoints=5000  SaveToWorkspace=off  SaveName=ss1_Pm2  YMin=0.99955  YMax=1  SampleTime=-1  DataFormat=Array
  128 MVA 13.8kV 3600 rpm2 : powerlib/Machines/Synchronous Machine pu Standard  PresetModel=No  MechanicalLoad=Mechanical power Pm  ShowDetailedParameters=on  RotorType=Round  Units=per unit standard parameters  MeasurementBus=off  NominalParameters="[ 128e6  13.8e3   60 ]"  Reactances1=[ 1.68, 0.232064, 0.1536, 1.609984, 0.32, 0.2176, 0.094976 ]  Reactances2="[ 1.305, 0.296, 0.252, 0.474,  0.243,  0.18 ]"  dAxisTimeConstants=Open-circuit  qAxisTimeConstants=Open-circuit  TimeConstants1="[ 4.4849  0.0681  0.1  ]"  TimeConstants2="[ 5.89, 0.05,  0.6, 0.05 ]"  TimeConstants3="[  4.49  0.0681  0.0513  ]"  TimeConstants4=[ 8.0, 0.03, 0.3371, 0.0295 ]  TimeConstants5=[ 1.01, 0.053, 0.1 ]  TimeConstants6=[ 1.3201, 0.023, 1.0, 0.07 ]  TimeConstants7="[  1.01  0.053  0.051266  ]"  TimeConstants8=[ 1.3201, 0.0231, 0.3371, 0.0295 ]  StatorResistance=0.000125  Mechanical="[ 3.01  0 1 ]"  PolePairs=1  InitialConditions=[0 -35.8791 0.653244 0.653244 0.653244 11.9635 -108.037 131.963 1.40212]  SetSaturation=off  Saturation=[0.6404,0.7127,0.8441,0.9214,0.9956,1.082,1.19,1.316,1.457;0.7,0.7698,0.8872,0.9466,0.9969,1.046,1.1,1.151,1.201]  LoadFlowParameters=[1 85000000 0 0 0]  TsPowergui=0  TsBlock=-1  IterativeModel=Trapezoidal non iterative  IterativeDiscreteModel=Trapezoidal non iterative  BusType=PV  Pref=85e6  Qref=0  Qmin=-Inf  Qmax=Inf  PLF=0  QLF=0
  Bus Selector3 : BusSelector  OutputSignals="Output active power   Peo (pu),Output reactive power  Qeo (pu),dq0 components.Stator voltage  vd (pu),dq0 components.Stator voltage  vq (pu),Mechanical.Rotor angle deviation  d_theta (rad),Mechanical.Rotor speed  wm  (pu),Mechanical.Rotor speed deviation  dw (pu)"
  Constant1 : Constant
  Excitation System2 : sps_avr/Excitation System  tr=20e-3  reg=[ 200, 0.02 ]  exc=[ 1, 0 ]  tgr=[ 12.0, 1.0 ]  damp=[ 0.03, 1.0 ]  sat=[ 0, 0 ]  lim=[ -10.0, 10.0, 0 ]  v0=[1.025 1.4021]
  Gain : Gain  Gain=128e6
  Gain1 : Gain  Gain=128e6
  Ground2 : Ground
  Pref2 : Constant  Value=0.66406
  Steam Turbine and Governor1 : powerlib/Machines/Steam Turbine and Governor  gentype=Tandem-compound (single mass)  reg1="[ 1  0.05    0 ]"  reg2="[ 0.001  0.1 ]"  reg3="[ -10.0 0.1   0.1 1.0 ]"  N=3600  turb1="[ 0.12  0.13  10.0   0.32   ]"  turb2="[ 0.48   0.25   0  0.27 ]"  HA="[  1.5498   0.24894  0  0 ]"  KA="[  83.47  42.702  0  0 ]"  DA="[  0.3104  0.05  0  0 ]*8"  ini1=0.66412  ini2=[1.88924e-008,-120.067]
  Subsystem1 : Subsystem
  Terminator1 : Terminator
  Turbine1 : Scope  NumInputPorts=2
      settings: TimeRange=0.5  MaxDataPoints=5000  SaveToWorkspace=off  SaveName=ss1_ScopeData2  YMin=-3e-07~-1  YMax=5e-08~1  SampleTime=-1
  Va Gen : Scope
      settings: TimeRange=0.007300652369719236  TickLabels=on  MaxDataPoints=5000  SaveToWorkspace=off  SaveName=ss1_vf4  YMin=-15000  YMax=15000  SampleTime=-1  DataFormat=Array
  Va4 : powerlib/Measurements/Voltage Measurement  Tag=PoWeRsYsTeMmEaSuReMeNt  PhasorSimulation=off  OutputType=Magnitude  PSBequivalent=0
  Vref2 : Constant  Value=1.025
  output Ground5 : powerlib/Elements/Ground  LConnTagsString=a
  A : PMIOPort  Port=1  Side=Right
  B : PMIOPort  Port=2  Side=Right
  C : PMIOPort  Port=3  Side=Right
  tag scope: ss1_OmegaGen_3=global, ss1_Pgen_3=global, ss1_Qgen_3=global
  wires:
  Constant1/1 -> Steam Turbine and Governor1/1
  Bus Selector3/5 -> Steam Turbine and Governor1/4  "<Rotor angle deviation  d_theta (rad)>"
  Subsystem1/2(T_23) -> Turbine1/2  "T2 (Gen-LP)  T3(LP-HP)  [pu]"
  Steam Turbine and Governor1/3 -> Terminator1/1
  Bus Selector3/7 -> Subsystem1/1(In1)  "<Rotor speed deviation  dw (pu)>"
  Vref2/1 -> Excitation System2/1
  Pref2/1 -> Steam Turbine and Governor1/2
  Steam Turbine and Governor1/1 -> Subsystem1/2(In2)
  Subsystem1/1(dw_123) -> Turbine1/1  "dw1(Gen)  dw2(LP)   dw3(HP) [pu]"
  Steam Turbine and Governor1/4 -> 128 MVA 13.8kV 3600 rpm2/1
  Steam Turbine and Governor1/2 -> Subsystem1/3(In3)
  Bus Selector3/6 -> [ss1_OmegaGen_3], " Speed (pu)2"/1, Steam Turbine and Governor1/3  "<Rotor speed  wm  (pu)>"
  128 MVA 13.8kV 3600 rpm2/1 -> Bus Selector3/1
  Ground2/1 -> Excitation System2/4
  Bus Selector3/4 -> Excitation System2/3  "<Stator voltage  vq (pu)>"
  Bus Selector3/3 -> Excitation System2/2  "<Stator voltage  vd (pu)>"
  Excitation System2/1 -> 128 MVA 13.8kV 3600 rpm2/2
  Va4/1 -> Va Gen/1
  Gain/1 -> [ss1_Pgen_3]
  Bus Selector3/1 -> Gain/1  "<Output active power   Peo (pu)>"
  Gain1/1 -> [ss1_Qgen_3]
  Bus Selector3/2 -> Gain1/1  "<Output reactive power  Qeo (pu)>"
  connections:
  output Ground5/LConn1 -- Va4/LConn2
  C/RConn1 -- 128 MVA 13.8kV 3600 rpm2/RConn3
  128 MVA 13.8kV 3600 rpm2/RConn2 -- B/RConn1
  Va4/LConn1 -- 128 MVA 13.8kV 3600 rpm2/RConn1 -- A/RConn1

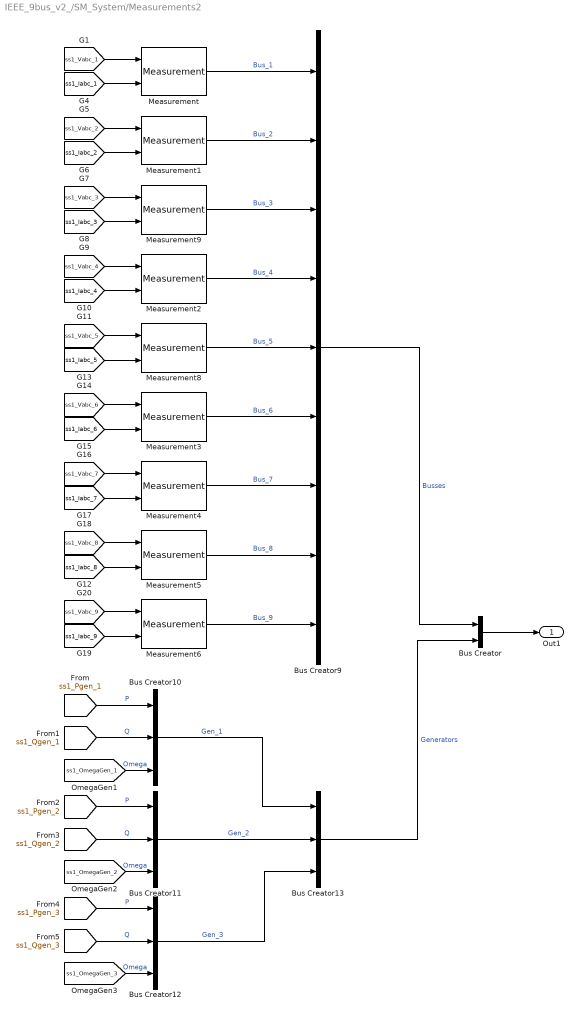
== system IEEE_9bus_v2_/SM_System/Measurements2 ==
  Bus Creator : BusCreator  Inputs=2
  Bus Creator{10..13} (4 alike) : BusCreator  Inputs=3
  Bus Creator9 : BusCreator  Inputs=9
  Measurement : library/Measurement  Vnom=16500
  Measurement1 : library/Measurement  Vnom=18000
  Measurement{2..6,8} (6 alike) : library/Measurement  Vnom=230000
  Measurement9 : library/Measurement  Vnom=13800
  Out1 : Outport
  wires:
  [ss1_Pgen_2] -> Bus Creator11/1  "P"
  [ss1_Qgen_3] -> Bus Creator12/2  "Q"
  [ss1_Qgen_2] -> Bus Creator11/2  "Q"
  [ss1_Qgen_1] -> Bus Creator10/2  "Q"
  [ss1_Pgen_1] -> Bus Creator10/1  "P"
  [ss1_OmegaGen_1] -> Bus Creator10/3  "Omega"
  [ss1_OmegaGen_2] -> Bus Creator11/3  "Omega"
  [ss1_Pgen_3] -> Bus Creator12/1  "P"
  [ss1_OmegaGen_3] -> Bus Creator12/3  "Omega"
  Bus Creator9/1 -> Bus Creator/1  "Busses"
  Bus Creator13/1 -> Bus Creator/2  "Generators"
  Bus Creator10/1 -> Bus Creator13/1  "Gen_1"
  Bus Creator11/1 -> Bus Creator13/2  "Gen_2"
  Bus Creator12/1 -> Bus Creator13/3  "Gen_3"
  Bus Creator/1 -> Out1/1
  [ss1_Vabc_1] -> Measurement/1
  [ss1_Iabc_1] -> Measurement/2
  Measurement/1 -> Bus Creator9/1  "Bus_1"
  [ss1_Iabc_2] -> Measurement1/2
  [ss1_Vabc_2] -> Measurement1/1
  [ss1_Vabc_3] -> Measurement9/1
  [ss1_Iabc_3] -> Measurement9/2
  [ss1_Vabc_4] -> Measurement2/1
  [ss1_Iabc_4] -> Measurement2/2
  [ss1_Iabc_5] -> Measurement8/2
  [ss1_Vabc_5] -> Measurement8/1
  [ss1_Vabc_6] -> Measurement3/1
  [ss1_Iabc_6] -> Measurement3/2
  [ss1_Iabc_9] -> Measurement6/2
  [ss1_Vabc_7] -> Measurement4/1
  [ss1_Iabc_7] -> Measurement4/2
  [ss1_Vabc_8] -> Measurement5/1
  [ss1_Iabc_8] -> Measurement5/2
  [ss1_Vabc_9] -> Measurement6/1
  Measurement6/1 -> Bus Creator9/9  "Bus_9"
  Measurement1/1 -> Bus Creator9/2  "Bus_2"
  Measurement9/1 -> Bus Creator9/3  "Bus_3"
  Measurement2/1 -> Bus Creator9/4  "Bus_4"
  Measurement8/1 -> Bus Creator9/5  "Bus_5"
  Measurement3/1 -> Bus Creator9/6  "Bus_6"
  Measurement4/1 -> Bus Creator9/7  "Bus_7"
  Measurement5/1 -> Bus Creator9/8  "Bus_8"

== system IEEE_9bus_v2_/SM_System/OPMonitor ==
  Mux8 : Mux  Inputs=3
  OpMonitor : rtlab/Monitoring/OpMonitor  compute_time=on  real_step=on  idle_time=off  nb_overruns=on  user_time=off  user_name=my_event_name,another_event_name
  Monitor : Outport
  wires:
  OpMonitor/1 -> Mux8/2
  OpMonitor/2 -> Mux8/3
  OpMonitor/3 -> Mux8/1
  Mux8/1 -> Monitor/1

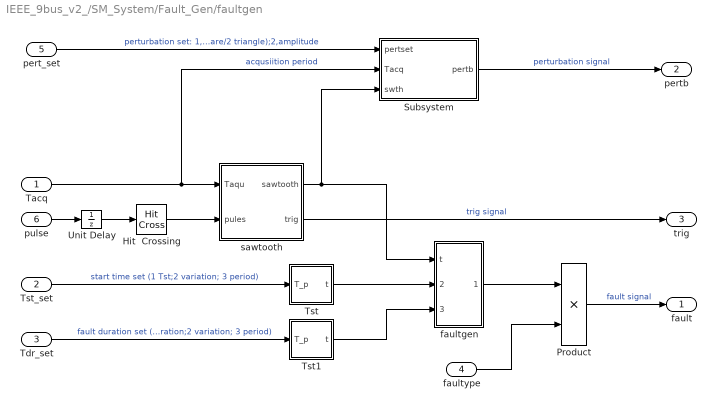
== system IEEE_9bus_v2_/SM_System/Fault_Gen/faultgen ==
  Tacq : Inport
  Tst_set : Inport  Port=2
  Tdr_set : Inport  Port=3
  faultype : Inport  Port=4
  pert_set : Inport  Port=5
  pulse : Inport  Port=6
  Hit  Crossing : HitCross  HitCrossingDirection=rising  SampleTime=Ts
  Product : Product  SampleTime=Ts  RndMeth=Zero
  Subsystem : Subsystem
  Tst : Subsystem
  Tst1 : Subsystem
  Unit Delay : UnitDelay  SampleTime=Ts
  faultgen : Subsystem
  sawtooth : Subsystem
  fault : Outport  SampleTime=Ts
  pertb : Outport  Port=2
  trig : Outport  Port=3
  wires:
  sawtooth/1(sawtooth) -> Subsystem/3(swth), faultgen/1(t)
  Tst/1(t) -> faultgen/2(Tstat)
  Tst1/1(t) -> faultgen/3(Tdur)
  Tacq/1 -> Subsystem/2(Tacq), sawtooth/1(Taqu)  "acqusiition period"
  pert_set/1 -> Subsystem/1(pertset)  "perturbation set: 1,(0 none/1 square/2 triangle);2,amplitude"
  Subsystem/1(pertb) -> pertb/1  "perturbation signal"
  sawtooth/2(trig) -> trig/1  "trig signal"
  Tst_set/1 -> Tst/1(T_p)  "start time set (1 Tst;2 variation; 3 period)"
  Tdr_set/1 -> Tst1/1(T_p)  "fault duration set (1 duration;2 variation; 3 period)"
  Hit  Crossing/1 -> sawtooth/2(pules)
  pulse/1 -> Unit Delay/1
  faultgen/1(fault) -> Product/1
  faultype/1 -> Product/2
  Product/1 -> fault/1  "fault signal"
  Unit Delay/1 -> Hit  Crossing/1

== system IEEE_9bus_v2_/SM_System/Generator BUS1x1/Subsystem1 ==
  In1 : Inport
  In2 : Inport  Port=2
  In3 : Inport  Port=3
  Gain : Gain  Gain=-1  SaturateOnIntegerOverflow=on  OutDataTypeStr=Inherit: Same as input  ParamDataTypeStr=Inherit: Same as input
  Mux : Mux  Inputs=2
  Selector : Selector  InputPortWidth=4  IndexOptions=Index vector (dialog)  Indices=[4 3]  OutputSizes=1
  Selector1 : Selector  InputPortWidth=4  IndexOptions=Index vector (dialog)  Indices=[4 3]  OutputSizes=1
  dw_123 : Outport
  T_23 : Outport  Port=2
  wires:
  Selector/1 -> Mux/2
  Mux/1 -> dw_123/1
  In1/1 -> Mux/1
  In2/1 -> Selector/1
  In3/1 -> Selector1/1
  Selector1/1 -> Gain/1
  Gain/1 -> T_23/1

== system IEEE_9bus_v2_/SM_System/Generator BUS2x1/Subsystem1 ==
  In1 : Inport
  In2 : Inport  Port=2
  In3 : Inport  Port=3
  Gain : Gain  Gain=-1  SaturateOnIntegerOverflow=on  OutDataTypeStr=Inherit: Same as input  ParamDataTypeStr=Inherit: Same as input
  Mux : Mux  Inputs=2
  Selector : Selector  InputPortWidth=4  IndexOptions=Index vector (dialog)  Indices=[4 3]  OutputSizes=1
  Selector1 : Selector  InputPortWidth=4  IndexOptions=Index vector (dialog)  Indices=[4 3]  OutputSizes=1
  dw_123 : Outport
  T_23 : Outport  Port=2
  wires:
  Selector/1 -> Mux/2
  Mux/1 -> dw_123/1
  In1/1 -> Mux/1
  In2/1 -> Selector/1
  In3/1 -> Selector1/1
  Selector1/1 -> Gain/1
  Gain/1 -> T_23/1

== system IEEE_9bus_v2_/SM_System/Generator BUS3x1/Subsystem1 ==
  In1 : Inport
  In2 : Inport  Port=2
  In3 : Inport  Port=3
  Gain : Gain  Gain=-1  SaturateOnIntegerOverflow=on  OutDataTypeStr=Inherit: Same as input  ParamDataTypeStr=Inherit: Same as input
  Mux : Mux  Inputs=2
  Selector : Selector  InputPortWidth=4  IndexOptions=Index vector (dialog)  Indices=[4 3]  OutputSizes=1
  Selector1 : Selector  InputPortWidth=4  IndexOptions=Index vector (dialog)  Indices=[4 3]  OutputSizes=1
  dw_123 : Outport
  T_23 : Outport  Port=2
  wires:
  Selector/1 -> Mux/2
  Mux/1 -> dw_123/1
  In1/1 -> Mux/1
  In2/1 -> Selector/1
  In3/1 -> Selector1/1
  Selector1/1 -> Gain/1
  Gain/1 -> T_23/1

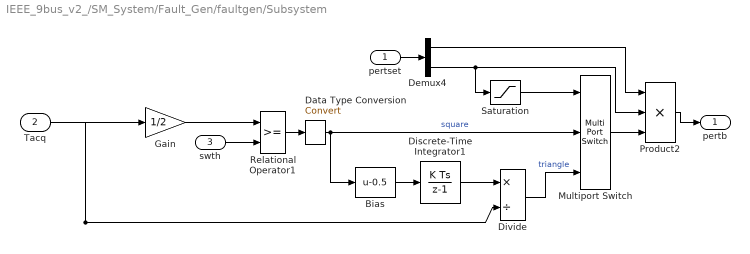
== system IEEE_9bus_v2_/SM_System/Fault_Gen/faultgen/Subsystem ==
  pertset : Inport
  Tacq : Inport  Port=2
  swth : Inport  Port=3
  Bias : Bias  Bias=-0.5
  Data Type Conversion : DataTypeConversion
  Demux4 : Demux  Outputs=2
  Discrete-Time Integrator1 : DiscreteIntegrator  gainval=2  SampleTime=Ts  LimitOutput=on  LowerSaturationLimit=0  ICPrevOutput=DiscIntNeverNeededParam  ICPrevScaledInput=DiscIntNeverNeededParam
  Divide : Product  Inputs=*/
  Gain : Gain  Gain=1/2
  Multiport Switch : MultiPortSwitch  Inputs=2
  Product2 : Product  Inputs=3  RndMeth=Zero
  Relational Operator1 : RelationalOperator  OutDataTypeStr=boolean
  Saturation : Saturate  UpperLimit=2  LowerLimit=1
  pertb : Outport
  wires:
  Gain/1 -> Relational Operator1/1
  Relational Operator1/1 -> Data Type Conversion/1
  Bias/1 -> Discrete-Time Integrator1/1
  Data Type Conversion/1 -> Bias/1, Multiport Switch/2  "square"
  Discrete-Time Integrator1/1 -> Divide/1
  Saturation/1 -> Multiport Switch/1
  Divide/1 -> Multiport Switch/3  "triangle"
  Multiport Switch/1 -> Product2/3
  Demux4/1 -> Product2/1
  Demux4/2 -> Saturation/1, Product2/2
  swth/1 -> Relational Operator1/2
  Tacq/1 -> Gain/1, Divide/2
  pertset/1 -> Demux4/1
  Product2/1 -> pertb/1

== system IEEE_9bus_v2_/SM_System/Fault_Gen/faultgen/Tst ==
  note: Prevents division by 0 at initial step
      | if a delay 1/Z is used before hand
  T_p : Inport
  Add : Sum
  Demux : Demux  Outputs=3
  Discrete-Time Integrtor : DiscreteIntegrator  ExternalReset=rising  SampleTime=-1  ICPrevOutput=DiscIntNeverNeededParam  ICPrevScaledInput=DiscIntNeverNeededParam
  Divide : Product  Inputs=*/
  Memory : Memory
  Relational Operator : RelationalOperator  OutDataTypeStr=boolean
  Saturation : Saturate  UpperLimit=inf  LowerLimit=0.0001
  t : Outport
  wires:
  Relational Operator/1 -> Discrete-Time Integrtor/2
  Memory/1 -> Relational Operator/1
  Discrete-Time Integrtor/1 -> Add/2, Memory/1
  Divide/1 -> Discrete-Time Integrtor/1
  T_p/1 -> Demux/1
  Demux/1 -> Add/1
  Demux/2 -> Divide/1, Relational Operator/2
  Add/1 -> t/1
  Demux/3 -> Saturation/1
  Saturation/1 -> Divide/2

== system IEEE_9bus_v2_/SM_System/Fault_Gen/faultgen/Tst1 ==
  note: Prevents division by 0 at initial step
      | if a delay 1/Z is used before hand
  T_p : Inport
  Add : Sum
  Demux : Demux  Outputs=3
  Discrete-Time Integrtor : DiscreteIntegrator  ExternalReset=rising  SampleTime=-1  ICPrevOutput=DiscIntNeverNeededParam  ICPrevScaledInput=DiscIntNeverNeededParam
  Divide : Product  Inputs=*/
  Memory : Memory
  Relational Operator : RelationalOperator  OutDataTypeStr=boolean
  Saturation : Saturate  UpperLimit=inf  LowerLimit=0.0001
  t : Outport
  wires:
  Relational Operator/1 -> Discrete-Time Integrtor/2
  Memory/1 -> Relational Operator/1
  Discrete-Time Integrtor/1 -> Add/2, Memory/1
  Divide/1 -> Discrete-Time Integrtor/1
  T_p/1 -> Demux/1
  Demux/1 -> Add/1
  Demux/2 -> Divide/1, Relational Operator/2
  Add/1 -> t/1
  Demux/3 -> Saturation/1
  Saturation/1 -> Divide/2

== system IEEE_9bus_v2_/SM_System/Fault_Gen/faultgen/faultgen ==
  t : Inport
  Tstat : Inport  Port=2
  Tdur : Inport  Port=3
  Add : Sum
  Logical Operator : Logic  AllPortsSameDT=off  OutDataTypeStr=boolean
  Relational Operator1 : RelationalOperator  Operator=<=  OutDataTypeStr=boolean
  Relational Operatr : RelationalOperator  OutDataTypeStr=boolean
  fault : Outport
  wires:
  Add/1 -> Relational Operator1/2
  Relational Operator1/1 -> Logical Operator/2
  Relational Operatr/1 -> Logical Operator/1
  t/1 -> Relational Operatr/1, Relational Operator1/1
  Logical Operator/1 -> fault/1
  Tdur/1 -> Add/2
  Tstat/1 -> Relational Operatr/2, Add/1

== system IEEE_9bus_v2_/SM_System/Fault_Gen/faultgen/sawtooth ==
  Taqu : Inport
  pules : Inport  Port=2
  Constant : Constant
  Data Type Conversion : DataTypeConversion
  Discrete-Time Integrator : DiscreteIntegrator  ExternalReset=rising  SampleTime=Ts  ICPrevOutput=DiscIntNeverNeededParam  ICPrevScaledInput=DiscIntNeverNeededParam
  Logical Operator : Logic  AllPortsSameDT=off
  Memory : Memory
  Relational Operator : RelationalOperator  OutDataTypeStr=boolean
  Voltage and Current Bus1 : Scope  NumInputPorts=2
      settings: TimeRange=1  MaxDataPoints=15000  SaveToWorkspace=off  SaveName=mach8  YMin=0.0625~-1  YMax=0.1~1  SampleTime=-1
  sawtooth : Outport
  trig : Outport  Port=2
  wires:
  Constant/1 -> Discrete-Time Integrator/1
  Discrete-Time Integrator/1 -> Memory/1, sawtooth/1, Voltage and Current Bus1/1
  Memory/1 -> Relational Operator/1
  Logical Operator/1 -> Discrete-Time Integrator/2, Data Type Conversion/1
  Relational Operator/1 -> Logical Operator/2
  pules/1 -> Logical Operator/1
  Taqu/1 -> Relational Operator/2
  Data Type Conversion/1 -> trig/1
